simulink subsystem "StatePropagation"  (R2022a)
settings: Solver=VariableStepAuto  StartTime=0.0  StopTime=10.0  RelTol=1e-3
model mask{spaceRobot=spaceRobot, q_0=0, q_dot_0=0}
  mask prompts: q_0 "Config"; q_dot_0 "Speed"
undefined symbols (not defined in the file): n
settings Model: Creator=charl  LastModifiedBy=charl

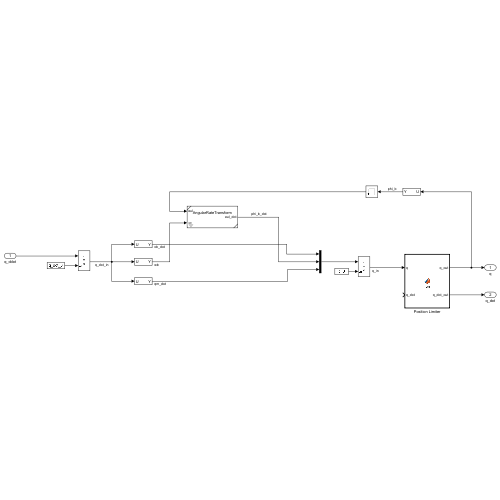
[thumbnail: Simulink's stored preview of the top-level diagram]
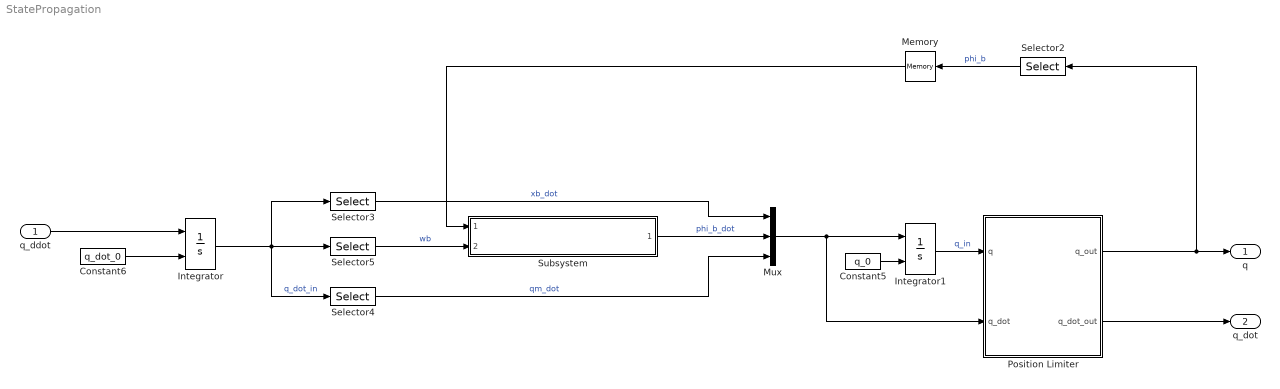
== system StatePropagation ==
  q_ddot : Inport
  Constant5 : Constant  Value=q_0
  Constant6 : Constant  Value=q_dot_0
  Integrator : Integrator  InitialConditionSource=external
  Integrator1 : Integrator  InitialConditionSource=external
  Memory : Memory
  Mux : Mux  Inputs=3
  Position Limiter : MATLAB Function  TreatAsAtomicUnit=on
  Selector2 : Selector  IndexOptions=Index vector (dialog)  Indices=[4:6]  OutputSizes=1
  Selector3 : Selector  IndexOptions=Index vector (dialog)  Indices=[1:3]  OutputSizes=1
  Selector4 : Selector  IndexOptions=Index vector (dialog)  Indices=[7:6+n]  OutputSizes=1
  Selector5 : Selector  IndexOptions=Index vector (dialog)  Indices=[4:6]  OutputSizes=1
  Subsystem : Subsystem  ReferencedSubsystem=AngularRateTransform
  q : Outport
  q_dot : Outport  Port=2
  wires:
  Memory/1 -> Subsystem/1
  Mux/1 -> Position Limiter/2(q_dot), Integrator1/1
  Selector5/1 -> Subsystem/2  "wb"
  Selector4/1 -> Mux/3  "qm_dot"
  Selector3/1 -> Mux/1  "xb_dot"
  Subsystem/1 -> Mux/2  "phi_b_dot"
  Selector2/1 -> Memory/1  "phi_b"
  Integrator1/1 -> Position Limiter/1(q)  "q_in"
  Constant5/1 -> Integrator1/2
  Integrator/1 -> Selector4/1, Selector5/1, Selector3/1  "q_dot_in"
  Constant6/1 -> Integrator/2
  q_ddot/1 -> Integrator/1
  Position Limiter/1(q_out) -> q/1, Selector2/1
  Position Limiter/2(q_dot_out) -> q_dot/1

== matlab function StatePropagation/Position Limiter ==
  data: q input; q_out output; q_dot input; q_dot_out output; jointLims parameter
function [q_out, q_dot_out] = fcn(q, q_dot, jointLims)

q_out = q;  
q_dot_out = q_dot;

for i=7:6+size(jointLims, 1)
    lims = jointLims(i-6, :);


    if q(i) < lims(1)
        q_out(i) = lims(1);
        q_dot_out(i) = 0;

    elseif q(i) > lims(2)
        q_out(i) = lims(2);
        q_dot_out(i) = 0;
    end
end
